simulink model "DockingApproachExample_Ext"  (Simulink 8.7)
settings: Solver=FixedStepDiscrete  StartTime=0.0  StopTime=300  RelTol=1e-3
libraries: simulink x2
settings Model: Creator=mwwhalen  LastModifiedBy=hamza
settings DataIOCC: ExternalInput=[t,u]  SaveFormat=Dataset  SignalLoggingSaveFormat=ModelDataLogs
settings OptimizationCC: ExpressionDepthLimit=2147483647  InitFltsAndDblsToZero=on
settings DebuggingCC: SaveWithParameterizedLinksMsg=none  SignalResolutionControl=TryResolveAllWithWarning  SolverPrmCheckMsg=warning  MultiTaskDSMMsg=warning  MultiTaskCondExecSysMsg=none  FcnCallInpInsideContextMsg=UseLocalSettings  StateNameClashWarn=warning
settings SFSimCC: SimParseCustomCode=off
settings RTWCC: PackageGeneratedCodeAndArtifacts=on  PackageName=DockingApproachExample_Ext_Code.zip  RTWCompilerOptimization=on
settings GRTTargetCC: TargetFcnLib=ansi_tfl_tmw.mat  CombineOutputUpdateFcns=off  GRTInterface=on

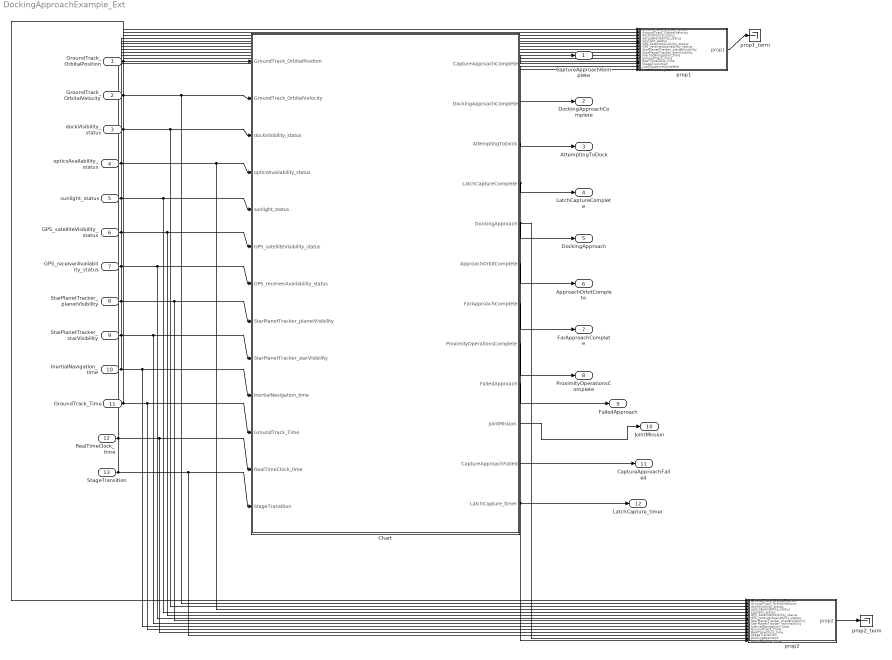
== system DockingApproachExample_Ext ==
  GroundTrack_OrbitalPosition : Inport
  GroundTrack_OrbitalVelocity : Inport  Port=2
  dockVisibility_status : Inport  Port=3
  opticsAvailability_status : Inport  Port=4
  sunlight_status : Inport  Port=5
  GPS_satelliteVisibility_status : Inport  Port=6
  GPS_receiverAvailability_status : Inport  Port=7
  StarPlanetTracker_planetVisibility : Inport  Port=8
  StarPlanetTracker_starVisibility : Inport  Port=9
  InertialNavigation_time : Inport  Port=10
  GroundTrack_Time : Inport  Port=11
  RealTimeClock_time : Inport  Port=12
  StageTransition : Inport  Port=13
  Chart : Stateflow chart  TreatAsAtomicUnit=on
  prop1 : Subsystem  TreatAsAtomicUnit=on  mask(Observer){AnnotationType=ensures, ObserverType=[]}
      mask prompts: AnnotationType "Type of annotation (pre/post...)"; ObserverType "Observer type"
      mask help:
      | Set an observer for the system.
      | The annotation type parameter sets the type of observer:
      | - requires : pre-condition
      | - ensures : post-condition
      | - assert : an assertion
      | - observer : the observer computes a special type of properties
      mask TypeOptions AnnotationType: ensures | requires | assert | observer
      mask Callback AnnotationType:
      | paramStr = get_param(gcb, 'MaskValues');
      | if strcmp(paramStr{1}(1),'o')
      | set_param(gcb,'MaskVisibilities',{'on';'on'});
      | paramStr{2} = 'ellipsoid';
      | set_param(gcb,'MaskValues',paramStr);
      | else
      | set_param(gcb,'MaskVisibilities',{'on';'off'});
      | end
      | clear paramStr;
      mask Callback ObserverType:
      | paramStr = get_param(gcb, 'MaskValues');
      | if strcmp(paramStr{1}(1),'o')
      | set_param(gcb,'MaskVisibilities',{'on';'on'});
      | paramStr{2} = 'ellipsoid';
      | set_param(gcb,'MaskValues',paramStr);
      | else
      | set_param(gcb,'MaskVisibilities',{'on';'off'});
      | end
      | clear paramStr;
      mask Display:
      | color('red')
      | text(0.5, 0.5, ['CoCoSpec: ''' get_param(gcb,'name') ''''], 'horizontalAlignment', 'center');
      | text(0.99, 0.03, '{\bf\fontsize{12}TO BE VERIFIED}', 'hor', 'right', 'ver', 'bottom', 'texmode', 'on');
  prop1_term : Terminator
  prop2 : Subsystem  TreatAsAtomicUnit=on  mask(Observer){AnnotationType=ensures, ObserverType=[]}
      mask prompts: AnnotationType "Type of annotation (pre/post...)"; ObserverType "Observer type"
      mask help:
      | Set an observer for the system.
      | The annotation type parameter sets the type of observer:
      | - requires : pre-condition
      | - ensures : post-condition
      | - assert : an assertion
      | - observer : the observer computes a special type of properties
      mask TypeOptions AnnotationType: ensures | requires | assert | observer
      mask Callback AnnotationType:
      | paramStr = get_param(gcb, 'MaskValues');
      | if strcmp(paramStr{1}(1),'o')
      | set_param(gcb,'MaskVisibilities',{'on';'on'});
      | paramStr{2} = 'ellipsoid';
      | set_param(gcb,'MaskValues',paramStr);
      | else
      | set_param(gcb,'MaskVisibilities',{'on';'off'});
      | end
      | clear paramStr;
      mask Callback ObserverType:
      | paramStr = get_param(gcb, 'MaskValues');
      | if strcmp(paramStr{1}(1),'o')
      | set_param(gcb,'MaskVisibilities',{'on';'on'});
      | paramStr{2} = 'ellipsoid';
      | set_param(gcb,'MaskValues',paramStr);
      | else
      | set_param(gcb,'MaskVisibilities',{'on';'off'});
      | end
      | clear paramStr;
      mask Display:
      | color('red')
      | text(0.5, 0.5, ['CoCoSpec: ''' get_param(gcb,'name') ''''], 'horizontalAlignment', 'center');
      | text(0.99, 0.03, '{\bf\fontsize{12}TO BE VERIFIED}', 'hor', 'right', 'ver', 'bottom', 'texmode', 'on');
  prop2_term : Terminator
  CaptureApproachComplete : Outport
  DockingApproachComplete : Outport  Port=2
  AttemptingToDock : Outport  Port=3
  LatchCaptureComplete : Outport  Port=4
  DockingApproach : Outport  Port=5
  ApproachOrbitComplete : Outport  Port=6
  FarApproachComplete : Outport  Port=7
  ProximityOperationsComplete : Outport  Port=8
  FailedApproach : Outport  Port=9
  JointMission : Outport  Port=10
  CaptureApproachFailed : Outport  Port=11
  LatchCapture_timer : Outport  Port=12
  wires:
  GroundTrack_OrbitalVelocity/1 -> Chart/2(GroundTrack_OrbitalVelocity), prop2/2(GroundTrack_OrbitalVelocity), prop1/2(GroundTrack_OrbitalVelocity)
  dockVisibility_status/1 -> Chart/3(dockVisibility_status), prop2/3(dockVisibility_status), prop1/3(dockVisibility_status)
  opticsAvailability_status/1 -> Chart/4(opticsAvailability_status), prop2/4(opticsAvailability_status), prop1/4(opticsAvailability_status)
  sunlight_status/1 -> Chart/5(sunlight_status), prop2/5(sunlight_status), prop1/5(sunlight_status)
  GPS_satelliteVisibility_status/1 -> Chart/6(GPS_satelliteVisibility_status), prop2/6(GPS_satelliteVisibility_status), prop1/6(GPS_satelliteVisibility_status)
  StarPlanetTracker_planetVisibility/1 -> Chart/8(StarPlanetTracker_planetVisibility), prop2/8(StarPlanetTracker_planetVisibility), prop1/8(StarPlanetTracker_planetVisibility)
  StarPlanetTracker_starVisibility/1 -> Chart/9(StarPlanetTracker_starVisibility), prop2/9(StarPlanetTracker_starVisibility), prop1/9(StarPlanetTracker_starVisibility)
  InertialNavigation_time/1 -> Chart/10(InertialNavigation_time), prop2/10(InertialNavigation_time), prop1/10(InertialNavigation_time)
  GroundTrack_Time/1 -> Chart/11(GroundTrack_Time), prop2/11(GroundTrack_Time), prop1/11(GroundTrack_Time)
  RealTimeClock_time/1 -> Chart/12(RealTimeClock_time), prop2/12(RealTimeClock_time), prop1/12(RealTimeClock_time)
  GroundTrack_OrbitalPosition/1 -> Chart/1(GroundTrack_OrbitalPosition), prop1/1(GroundTrack_OrbitalPosition), prop2/1(GroundTrack_OrbitalPosition)
  StageTransition/1 -> Chart/13(StageTransition), prop2/13(StageTransition), prop1/13(StageTransition)
  GPS_receiverAvailability_status/1 -> Chart/7(GPS_receiverAvailability_status), prop2/7(GPS_receiverAvailability_status), prop1/7(GPS_receiverAvailability_status)
  Chart/2(DockingApproachComplete) -> DockingApproachComplete/1
  Chart/1(CaptureApproachComplete) -> CaptureApproachComplete/1
  Chart/3(AttemptingToDock) -> AttemptingToDock/1
  Chart/4(LatchCaptureComplete) -> LatchCaptureComplete/1, prop1/14(LatchCaptureComplete)
  Chart/5(DockingApproach) -> DockingApproach/1, prop2/14(DockingApproach)
  Chart/6(ApproachOrbitComplete) -> ApproachOrbitComplete/1
  Chart/7(FarApproachComplete) -> FarApproachComplete/1
  Chart/8(ProximityOperationsComplete) -> ProximityOperationsComplete/1
  Chart/9(FailedApproach) -> FailedApproach/1
  Chart/10(JointMission) -> JointMission/1
  Chart/11(CaptureApproachFailed) -> CaptureApproachFailed/1
  Chart/12(LatchCapture_timer) -> LatchCapture_timer/1, prop1/15(LatchCapture_timer), prop2/15(LatchCapture_timer)
  prop1/1(prop1) -> prop1_term/1
  prop2/1(prop2) -> prop2_term/1

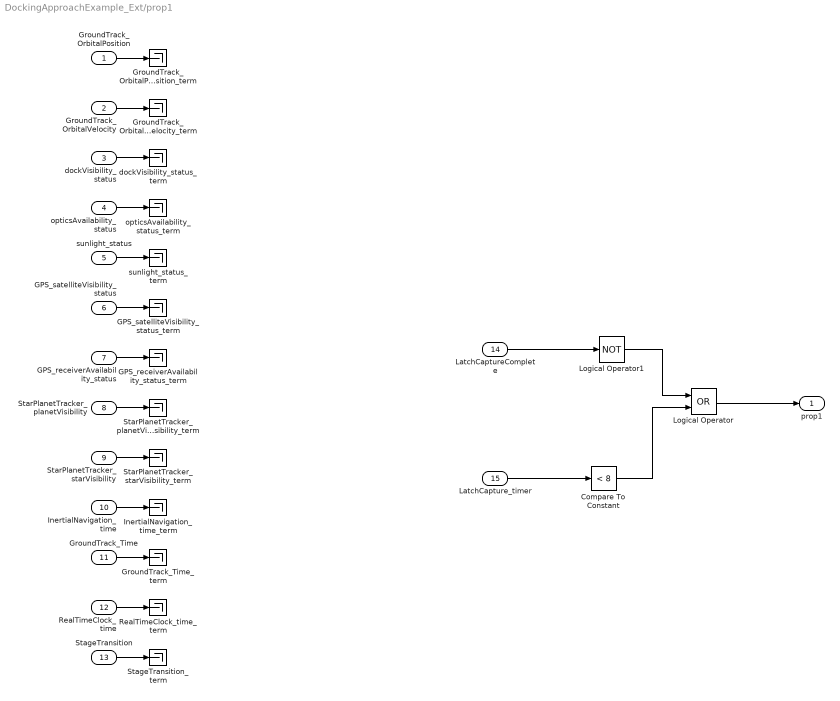
== system DockingApproachExample_Ext/prop1 ==
  GroundTrack_OrbitalPosition : Inport
  GroundTrack_OrbitalVelocity : Inport  Port=2
  dockVisibility_status : Inport  Port=3
  opticsAvailability_status : Inport  Port=4
  sunlight_status : Inport  Port=5
  GPS_satelliteVisibility_status : Inport  Port=6
  GPS_receiverAvailability_status : Inport  Port=7
  StarPlanetTracker_planetVisibility : Inport  Port=8
  StarPlanetTracker_starVisibility : Inport  Port=9
  InertialNavigation_time : Inport  Port=10
  GroundTrack_Time : Inport  Port=11
  RealTimeClock_time : Inport  Port=12
  StageTransition : Inport  Port=13
  LatchCaptureComplete : Inport  Port=14
  LatchCapture_timer : Inport  Port=15
  Compare To Constant : simulink/Logic and Bit Operations/Compare To Constant  relop=<  const=8  OutDataTypeStr=boolean
  GPS_receiverAvailability_status_term : Terminator
  GPS_satelliteVisibility_status_term : Terminator
  GroundTrack_OrbitalPosition_term : Terminator
  GroundTrack_OrbitalVelocity_term : Terminator
  GroundTrack_Time_term : Terminator
  InertialNavigation_time_term : Terminator
  Logical Operator : Logic  Operator=OR  AllPortsSameDT=off  OutDataTypeStr=boolean
  Logical Operator1 : Logic  Operator=NOT  AllPortsSameDT=off  OutDataTypeStr=boolean
  RealTimeClock_time_term : Terminator
  StageTransition_term : Terminator
  StarPlanetTracker_planetVisibility_term : Terminator
  StarPlanetTracker_starVisibility_term : Terminator
  dockVisibility_status_term : Terminator
  opticsAvailability_status_term : Terminator
  sunlight_status_term : Terminator
  prop1 : Outport
  wires:
  GroundTrack_OrbitalPosition/1 -> GroundTrack_OrbitalPosition_term/1
  GroundTrack_OrbitalVelocity/1 -> GroundTrack_OrbitalVelocity_term/1
  dockVisibility_status/1 -> dockVisibility_status_term/1
  opticsAvailability_status/1 -> opticsAvailability_status_term/1
  sunlight_status/1 -> sunlight_status_term/1
  GPS_satelliteVisibility_status/1 -> GPS_satelliteVisibility_status_term/1
  GPS_receiverAvailability_status/1 -> GPS_receiverAvailability_status_term/1
  StarPlanetTracker_planetVisibility/1 -> StarPlanetTracker_planetVisibility_term/1
  StarPlanetTracker_starVisibility/1 -> StarPlanetTracker_starVisibility_term/1
  InertialNavigation_time/1 -> InertialNavigation_time_term/1
  GroundTrack_Time/1 -> GroundTrack_Time_term/1
  RealTimeClock_time/1 -> RealTimeClock_time_term/1
  StageTransition/1 -> StageTransition_term/1
  LatchCaptureComplete/1 -> Logical Operator1/1
  LatchCapture_timer/1 -> Compare To Constant/1
  Logical Operator1/1 -> Logical Operator/1
  Compare To Constant/1 -> Logical Operator/2
  Logical Operator/1 -> prop1/1

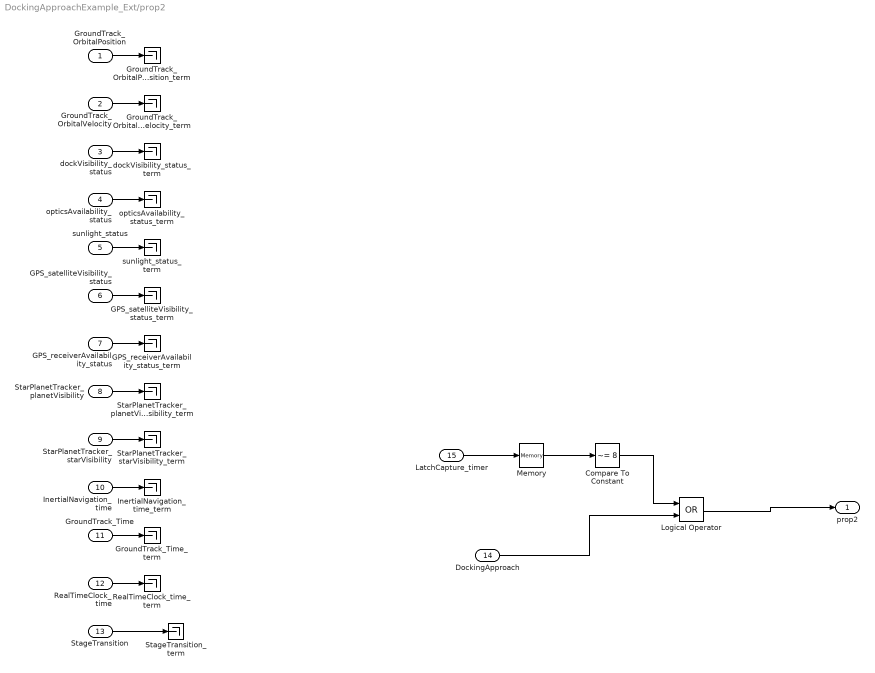
== system DockingApproachExample_Ext/prop2 ==
  GroundTrack_OrbitalPosition : Inport
  GroundTrack_OrbitalVelocity : Inport  Port=2
  dockVisibility_status : Inport  Port=3
  opticsAvailability_status : Inport  Port=4
  sunlight_status : Inport  Port=5
  GPS_satelliteVisibility_status : Inport  Port=6
  GPS_receiverAvailability_status : Inport  Port=7
  StarPlanetTracker_planetVisibility : Inport  Port=8
  StarPlanetTracker_starVisibility : Inport  Port=9
  InertialNavigation_time : Inport  Port=10
  GroundTrack_Time : Inport  Port=11
  RealTimeClock_time : Inport  Port=12
  StageTransition : Inport  Port=13
  DockingApproach : Inport  Port=14
  LatchCapture_timer : Inport  Port=15
  Compare To Constant : simulink/Logic and Bit Operations/Compare To Constant  relop=~=  const=8  OutDataTypeStr=boolean
  GPS_receiverAvailability_status_term : Terminator
  GPS_satelliteVisibility_status_term : Terminator
  GroundTrack_OrbitalPosition_term : Terminator
  GroundTrack_OrbitalVelocity_term : Terminator
  GroundTrack_Time_term : Terminator
  InertialNavigation_time_term : Terminator
  Logical Operator : Logic  Operator=OR  AllPortsSameDT=off  OutDataTypeStr=boolean
  Memory : Memory
  RealTimeClock_time_term : Terminator
  StageTransition_term : Terminator
  StarPlanetTracker_planetVisibility_term : Terminator
  StarPlanetTracker_starVisibility_term : Terminator
  dockVisibility_status_term : Terminator
  opticsAvailability_status_term : Terminator
  sunlight_status_term : Terminator
  prop2 : Outport
  wires:
  GroundTrack_OrbitalPosition/1 -> GroundTrack_OrbitalPosition_term/1
  GroundTrack_OrbitalVelocity/1 -> GroundTrack_OrbitalVelocity_term/1
  dockVisibility_status/1 -> dockVisibility_status_term/1
  opticsAvailability_status/1 -> opticsAvailability_status_term/1
  sunlight_status/1 -> sunlight_status_term/1
  GPS_satelliteVisibility_status/1 -> GPS_satelliteVisibility_status_term/1
  GPS_receiverAvailability_status/1 -> GPS_receiverAvailability_status_term/1
  StarPlanetTracker_planetVisibility/1 -> StarPlanetTracker_planetVisibility_term/1
  StarPlanetTracker_starVisibility/1 -> StarPlanetTracker_starVisibility_term/1
  InertialNavigation_time/1 -> InertialNavigation_time_term/1
  GroundTrack_Time/1 -> GroundTrack_Time_term/1
  RealTimeClock_time/1 -> RealTimeClock_time_term/1
  StageTransition/1 -> StageTransition_term/1
  DockingApproach/1 -> Logical Operator/2
  LatchCapture_timer/1 -> Memory/1
  Memory/1 -> Compare To Constant/1
  Compare To Constant/1 -> Logical Operator/1
  Logical Operator/1 -> prop2/1

== stateflow chart Chart ==
  settings: updateMethod=DISCRETE  sampleTime=1
  state fuel [parallel]
    settings: executionOrder=3
  state thrust [parallel]
    settings: executionOrder=2
    state y = compute(missionstate) [function]
      (default) -> (junction 74) : {}
    state y = command [function]
      (default) -> (junction 77) : {}
  state MissionPhaseStates [parallel]
    settings: executionOrder=1
    state FarApproach
    state JointStabilize
    state Start /
    state CollisionAvoidanceManuever/
      exit:
      ApproachOrbitComplete=0;
      ProximityOperationsComplete=0;
      FarApproachComplete=0;
      CaptureApproachComplete= 0;
    state FailedApproach /
      entry: FailedApproach=1;
    state ApproachOrbit
    state Disengage
    state ProximityOperations
    state JointMission /
      entry: JointMission=1;
    state DockingApproach/
      entry:
      DockingApproach = 1;
      DockingApproachComplete= 0;
      exit:
      DockingApproach = 0;
      state DockingApproach / [parallel]
        during :DockingApproach_timer = min(DockingApproach_timer+1,DockingApproach_timer_upper_limit/*9*/);
        settings: executionOrder=1
        note: This condition is our approximation
            | of missionState [GOOD]
        note: This condition is our approximation
            | of missionState [POOR]
        state StartApproach/
          entry : DockingApproach_timer = 0;
        state CheckTargetRelativeState
          /* missionState.compute (...) */
        state ReadyToDock/
          exit:
          DockingApproachComplete= 1;
        state ComputeThrust
        state DockingApproachFailed
        StartApproach -> CheckTargetRelativeState [order 1] : [dockingSensor_RelativePosition != NONE && ...
            | dockingSensor_RelativeVelocity != NONE && ...
            |  dockingSensor_RelativeAttitude != NONE &&...
            |  (DockingApproach_timer < DockingApproach_timer_upper_limit/*9*/)]
        (default) -> StartApproach
        StartApproach -> DockingApproachFailed [order 2] : [(DockingApproach_timer == DockingApproach_timer_upper_limit/*9*/)]
        CheckTargetRelativeState -> DockingApproachFailed [order 5] : [dockingSensor_targetState != GOOD]
        CheckTargetRelativeState -> DockingApproachFailed [order 4] : [dockingSensor_RelativePosition == NONE || ...
            | dockingSensor_RelativeVelocity == NONE || ...
            | dockingSensor_RelativeAttitude == NONE]
        CheckTargetRelativeState -> ReadyToDock [order 1] : [ dockingSensor_RelativePosition == GOOD &&...
            |   dockingSensor_RelativeVelocity == GOOD &...
            |   dockingSensor_RelativeAttitude == GOOD &&...
            |   dockingSensor_targetState == GOOD
            | /* MissionState_status == GOOD */ ]
        CheckTargetRelativeState -> DockingApproachFailed [order 3] : [(DockingApproach_timer == DockingApproach_timer_upper_limit/*9*/)]
        ComputeThrust -> CheckTargetRelativeState [order 1] : [thrust_status == EXIST && ...
            | fuel_status == GOOD]
        CheckTargetRelativeState -> ComputeThrust [order 2] : [ dockingSensor_RelativePosition == POOR &&...
            |   dockingSensor_RelativeVelocity == POOR &&...
            |   dockingSensor_RelativeAttitude == POOR &&...
            |   dockingSensor_targetState == POOR
            | /* MissionState_status == POOR */]
        ComputeThrust -> DockingApproachFailed [order 2] : [!(thrust_status == EXIST && ...
            |  fuel_status == GOOD)||...
            | DockingApproach_timer == DockingApproach_timer_upper_limit]
      state dockingSensor / [parallel]
        during:dockingSensor_timer = min(dockingSensor_timer + 1,dockingSensor_timer_upper_limit/*6*/);
        settings: executionOrder=2
        state Good /
          entry : dockingSensor_RelativePosition = GOOD;
          dockingSensor_RelativeVelocity = GOOD;
          dockingSensor_RelativeAttitude = GOOD;
          dockingSensor_targetState = GOOD;
          exit :  dockingSensor_timer = 0;
        state Poor /
          entry :dockingSensor_RelativePosition = POOR;
          dockingSensor_RelativeVelocity = POOR;
          dockingSensor_RelativeAttitude = POOR;
          dockingSensor_targetState = POOR;
        state Acquiring /
          entry : dockingSensor_RelativePosition = NONE;
          dockingSensor_RelativeVelocity = NONE;
          dockingSensor_RelativeAttitude = NONE;
          dockingSensor_targetState = NONE;
          exit :  dockingSensor_timer = 0;
        (default) -> MissionPhaseStates.DockingApproach.dockingSensor.Acquiring 
        Poor  -> MissionPhaseStates.DockingApproach.dockingSensor.Acquiring  [order 1] : [(dockingSensor_timer == dockingSensor_timer_upper_limit/*6*/) && ...
            | (dockVisibility_status == NONE || ...
            | opticsAvailability_status != AVAILABLE)]
        MissionPhaseStates.DockingApproach.dockingSensor.Acquiring  -> Poor  [order 1] : [dockVisibility_status != NONE && ...
            | opticsAvailability_status == AVAILABLE]
        MissionPhaseStates.DockingApproach.dockingSensor.Acquiring  -> MissionPhaseStates.DockingApproach.dockingSensor.Acquiring  [order 2] : [dockVisibility_status == NONE || ...
            | opticsAvailability_status != AVAILABLE]
        Poor  -> Poor  [order 3] : [(dockingSensor_timer < dockingSensor_timer_upper_limit/*6*/) &&...
            | (dockVisibility_status == NONE || ...
            | opticsAvailability_status != AVAILABLE)||...
            | (opticsAvailability_status == AVAILABLE &&...
            | (dockVisibility_status == POOR || ...
            | sunlight_status == BRIGHT))]
        Good  -> Poor  [order 1] : [(dockVisibility_status != GOOD && ...
            | opticsAvailability_status != AVAILABLE) || ...
            | sunlight_status == BRIGHT]
        Poor  -> Good  [order 2] : [(dockingSensor_timer < dockingSensor_timer_upper_limit) /* or ==6? */&&...
            | dockVisibility_status == GOOD && ...
            | opticsAvailability_status == AVAILABLE && ...
            | sunlight_status != BRIGHT]
        Good  -> Good  [order 2] : [dockVisibility_status == GOOD && ...
            | opticsAvailability_status == AVAILABLE && ...
            | sunlight_status != BRIGHT]
    state CaptureApproach /
      state CaptureApproach/ [parallel]
        during:CaptureApproach_timer = min(CaptureApproach_timer+1,CaptureApproach_timer_upper_limit)
        settings: executionOrder=1
        state StartApproach /
          entry :  CaptureApproach_timer = 0;
          CaptureApproachFailed = 0;
        state CheckOrbitalState
        state ComputeThrust /
          entry : /*thrust.compute(...
          CaptureMissionState)*/
        state OrientedForDockingApproach/
          exit:
          CaptureApproachComplete= 1;
        state CaptureApproachFailed /
          entry: CaptureApproachFailed = 1;
        (default) -> StartApproach 
        StartApproach  -> CheckOrbitalState [order 1] : [ OrbitalState_Position != NONE &&...
            |   OrbitalState_Velocity != NONE &&...
            |   OrbitalState_Attitude != NONE && ...
            |   OrbitalState_Time != NONE &&...
            |  (CaptureApproach_timer < CaptureApproach_timer_upper_limit)]
        StartApproach  -> CaptureApproachFailed  [order 2] : [CaptureApproach_timer ==...
            | CaptureApproach_timer_upper_limit]
        CheckOrbitalState -> OrientedForDockingApproach [order 1] : [OrbitalState_Position == GOOD...
            |  &&...
            |  OrbitalState_Velocity == GOOD...
            |  &&...
            |  OrbitalState_Attitude != NONE...
            |   &&...
            |  OrbitalState_Time == GOOD]
        ComputeThrust  -> CheckOrbitalState [order 1] : [thrust_status == EXIST &&...
            |  fuel_status == GOOD]
        CheckOrbitalState -> ComputeThrust  [order 2] : [OrbitalState_Position == POOR...
            |  &&...
            |  OrbitalState_Velocity == POOR...
            |  &&...
            |  OrbitalState_Attitude == NONE...
            |   &&...
            |  OrbitalState_Time == POOR]
        CheckOrbitalState -> CaptureApproachFailed  [order 3] : [(OrbitalState_Position == NONE ||...
            | OrbitalState_Velocity == NONE || ...
            | OrbitalState_Attitude == NONE ||...
            |  OrbitalState_Time == NONE) ||...
            |  (CaptureApproach_timer == ...
            | CaptureApproach_timer_upper_limit)]
        ComputeThrust  -> CaptureApproachFailed  [order 2] : [!(thrust_status == EXIST &&...
            | fuel_status == GOOD) || (CaptureApproach_timer == CaptureApproach_timer_upper_limit)]
      state OrbitalState_Active/ [parallel]
        settings: executionOrder=2
        state OrbitalState_Complex / [parallel]
          settings: executionOrder=1
          state OrbitalState/ [parallel]
            settings: executionOrder=1
            state Acquiring /
              entry : OrbitalState_Position = NONE;
              OrbitalState_Velocity = NONE;
              OrbitalState_Attitude = NONE;
            state POOR /
              entry : OrbitalState_Position = POOR;
              OrbitalState_Velocity = POOR;
              OrbitalState_Attitude = NONE;
            state pvGOOD /
              entry : OrbitalState_Position = GOOD;
              OrbitalState_Velocity = GOOD;
              OrbitalState_Attitude = POOR;
            state GOOD /
              entry : OrbitalState_Position = GOOD;
              OrbitalState_Velocity = GOOD;
              OrbitalState_Attitude = GOOD;
            MissionPhaseStates.CaptureApproach.OrbitalState_Active.OrbitalState_Complex.OrbitalState.Acquiring  -> MissionPhaseStates.CaptureApproach.OrbitalState_Active.OrbitalState_Complex.OrbitalState.Acquiring  [order 2] : [GPS_AbsolutePosition == NONE && GPS_AbsoluteVelocity == NONE && ...
                | StarPlanetTracker_AbsolutePosition == NONE && ...
                | StarPlanetTracker_AbsoluteVelocity == NONE &&...
                | GroundTrack_OrbitalPosition == NONE&&...
                | GroundTrack_OrbitalVelocity == NONE]
            (default) -> MissionPhaseStates.CaptureApproach.OrbitalState_Active.OrbitalState_Complex.OrbitalState.Acquiring 
            MissionPhaseStates.CaptureApproach.OrbitalState_Active.OrbitalState_Complex.OrbitalState.POOR  -> MissionPhaseStates.CaptureApproach.OrbitalState_Active.OrbitalState_Complex.OrbitalState.Acquiring  [order 1] : [(GroundTrack_OrbitalPosition == NONE &&...
                | GPS_AbsolutePosition == NONE &&...
                | StarPlanetTracker_AbsolutePosition == NONE) &&...
                | (GroundTrack_OrbitalVelocity == NONE &&...
                | GPS_AbsoluteVelocity == NONE &&...
                | StarPlanetTracker_AbsoluteVelocity == NONE)]
            MissionPhaseStates.CaptureApproach.OrbitalState_Active.OrbitalState_Complex.OrbitalState.Acquiring  -> MissionPhaseStates.CaptureApproach.OrbitalState_Active.OrbitalState_Complex.OrbitalState.POOR  [order 1] : [!(GPS_AbsolutePosition == NONE &&...
                |  StarPlanetTracker_AbsolutePosition == NONE&&...
                | GroundTrack_OrbitalPosition == NONE)&&...
                | !(GPS_AbsoluteVelocity == NONE &&...
                |  StarPlanetTracker_AbsoluteVelocity == NONE&&...
                | GroundTrack_OrbitalVelocity == NONE)]
            MissionPhaseStates.CaptureApproach.OrbitalState_Active.OrbitalState_Complex.OrbitalState.POOR  -> (junction 140) [order 2] : [((GroundTrack_OrbitalPosition == GOOD && ...
                |   GPS_AbsolutePosition == GOOD)|| ...
                |   (GroundTrack_OrbitalPosition == GOOD &&...
                | StarPlanetTracker_AbsolutePosition == GOOD)||...
                | (StarPlanetTracker_AbsolutePosition == GOOD &&...
                |  GPS_AbsolutePosition == GOOD)||...
                |  (InertialNavigation_AbsolutePosition == GOOD&&...
                |  GroundTrack_OrbitalPosition == GOOD)||...
                | (InertialNavigation_AbsolutePosition == GOOD&&...
                | GPS_AbsolutePosition == GOOD)|| ...
                | (InertialNavigation_AbsolutePosition == GOOD&&...
                |  StarPlanetTracker_AbsolutePosition == GOOD))]
            (junction 141) -> MissionPhaseStates.CaptureApproach.OrbitalState_Active.OrbitalState_Complex.OrbitalState.POOR  : [!((GroundTrack_OrbitalVelocity == GOOD && ...
                |   GPS_AbsoluteVelocity == GOOD)|| ...
                |   (GroundTrack_OrbitalVelocity == GOOD &&...
                | StarPlanetTracker_AbsoluteVelocity == GOOD)||...
                | (StarPlanetTracker_AbsoluteVelocity == GOOD &&...
                |  GPS_AbsoluteVelocity == GOOD)||...
                | (InertialNavigation_AbsoluteVelocity == GOOD&&...
                |  GroundTrack_OrbitalVelocity == GOOD)||...
                | (InertialNavigation_AbsoluteVelocity == GOOD&&...
                | GPS_AbsoluteVelocity == GOOD)|| ...
                | (InertialNavigation_AbsoluteVelocity == GOOD&&...
                |  StarPlanetTracker_AbsoluteVelocity == GOOD))]
            (junction 140) -> (junction 142) : [((GroundTrack_OrbitalVelocity == GOOD && ...
                |   GPS_AbsoluteVelocity == GOOD)|| ...
                |   (GroundTrack_OrbitalVelocity == GOOD &&...
                | StarPlanetTracker_AbsoluteVelocity == GOOD)||...
                | (StarPlanetTracker_AbsoluteVelocity == GOOD &&...
                |  GPS_AbsoluteVelocity == GOOD)||...
                | (InertialNavigation_AbsoluteVelocity == GOOD&&...
                |  GroundTrack_OrbitalVelocity == GOOD)||...
                | (InertialNavigation_AbsoluteVelocity == GOOD&&...
                | GPS_AbsoluteVelocity == GOOD)|| ...
                | (InertialNavigation_AbsoluteVelocity == GOOD&&...
                |  StarPlanetTracker_AbsoluteVelocity == GOOD))]
            (junction 143) -> (junction 141) : [!(InertialNavigation_AbsoluteAttitude == GOOD||...
                | StarPlanetTracker_AbsoluteAttitude == GOOD)]
            (junction 142) -> pvGOOD  : [InertialNavigation_AbsoluteAttitude == GOOD||...
                | StarPlanetTracker_AbsoluteAttitude == GOOD]
            MissionPhaseStates.CaptureApproach.OrbitalState_Active.OrbitalState_Complex.OrbitalState.GOOD  -> (junction 143) [order 1] : [!((GroundTrack_OrbitalPosition == GOOD && ...
                |   GPS_AbsolutePosition == GOOD)|| ...
                |   (GroundTrack_OrbitalPosition == GOOD &&...
                | StarPlanetTracker_AbsolutePosition == GOOD)||...
                | (StarPlanetTracker_AbsolutePosition == GOOD &&...
                |  GPS_AbsolutePosition == GOOD)||...
                |  (InertialNavigation_AbsolutePosition == GOOD&&...
                |  GroundTrack_OrbitalPosition == GOOD)||...
                | (InertialNavigation_AbsolutePosition == GOOD&&...
                | GPS_AbsolutePosition == GOOD)|| ...
                | (InertialNavigation_AbsolutePosition == GOOD&&...
                |  StarPlanetTracker_AbsolutePosition == GOOD))]
            pvGOOD  -> MissionPhaseStates.CaptureApproach.OrbitalState_Active.OrbitalState_Complex.OrbitalState.GOOD  : [(GroundTrack_OrbitalPosition == GOOD || ...
                | GPS_AbsolutePosition == GOOD || ...
                | StarPlanetTracker_AbsolutePosition == GOOD)...
                |  && (GroundTrack_OrbitalVelocity == GOOD || ...
                | GPS_AbsoluteVelocity == GOOD || ...
                | StarPlanetTracker_AbsoluteVelocity == GOOD)...
                | && StarPlanetTracker_AbsoluteAttitude == GOOD]/
                | /*send(callibrate,InertialNavigation)*/
            MissionPhaseStates.CaptureApproach.OrbitalState_Active.OrbitalState_Complex.OrbitalState.GOOD  -> MissionPhaseStates.CaptureApproach.OrbitalState_Active.OrbitalState_Complex.OrbitalState.GOOD  [order 2] : [(GroundTrack_OrbitalPosition == GOOD || ...
                | GPS_AbsolutePosition == GOOD || ...
                | StarPlanetTracker_AbsolutePosition == GOOD)...
                |  && (GroundTrack_OrbitalVelocity == GOOD || ...
                | GPS_AbsoluteVelocity == GOOD || ...
                | StarPlanetTracker_AbsoluteVelocity == GOOD)...
                | && StarPlanetTracker_AbsoluteAttitude == GOOD]/
                | /*send(callibrate,InertialNavigation)*/
          state y = RealTimeClock_callibrate [function]
            (default) -> (junction 157) : {}
          state OrbitalState2 / [parallel]
            settings: executionOrder=2
            state POOR/
              entry : OrbitalState_Time = POOR
            state GOOD /
              entry : OrbitalState_Time = GOOD
            (default) -> MissionPhaseStates.CaptureApproach.OrbitalState_Active.OrbitalState_Complex.OrbitalState2.POOR
            MissionPhaseStates.CaptureApproach.OrbitalState_Active.OrbitalState_Complex.OrbitalState2.GOOD  -> MissionPhaseStates.CaptureApproach.OrbitalState_Active.OrbitalState_Complex.OrbitalState2.POOR [order 1] : [RealTimeClock_time != GOOD]
            MissionPhaseStates.CaptureApproach.OrbitalState_Active.OrbitalState_Complex.OrbitalState2.POOR -> MissionPhaseStates.CaptureApproach.OrbitalState_Active.OrbitalState_Complex.OrbitalState2.GOOD  : [GroundTrack_Time== GOOD...
                | || GPS_AbsoluteTime == GOOD || ...
                | StarPlanetTracker_AbsoluteTime == GOOD]
            MissionPhaseStates.CaptureApproach.OrbitalState_Active.OrbitalState_Complex.OrbitalState2.GOOD  -> MissionPhaseStates.CaptureApproach.OrbitalState_Active.OrbitalState_Complex.OrbitalState2.GOOD  [order 2] : [GroundTrack_Time == GOOD...
                | || GPS_AbsoluteTime == GOOD || ...
                | StarPlanetTracker_AbsoluteTime == GOOD]...
                | /*/RealTimeClock_callibrate()*/
        state GPS / [parallel]
          during:GPS_timer = min(GPS_timer + 1,GPS_timer_upper_limit/*6*/);
          settings: executionOrder=2
          state ACQUIRING /
            entry : GPS_AbsolutePosition = NONE;
            GPS_AbsoluteVelocity = NONE;
            GPS_AbsoluteTime = NONE;
          state POOR /
            entry : GPS_timer = 0;
            GPS_AbsolutePosition = POOR;
            GPS_AbsoluteVelocity = POOR;
            GPS_AbsoluteTime = POOR;
          state GOOD /
            entry : GPS_AbsolutePosition = GOOD;
            GPS_AbsoluteVelocity = GOOD;
            GPS_AbsoluteTime = GOOD;
          MissionPhaseStates.CaptureApproach.OrbitalState_Active.GPS.POOR  -> MissionPhaseStates.CaptureApproach.OrbitalState_Active.GPS.ACQUIRING  [order 1] : [(GPS_timer == GPS_timer_upper_limit /*5*/) && (GPS_satelliteVisibility_status == NONE || ...
              | GPS_receiverAvailability_status != AVAILABLE)]
          (default) -> MissionPhaseStates.CaptureApproach.OrbitalState_Active.GPS.ACQUIRING 
          MissionPhaseStates.CaptureApproach.OrbitalState_Active.GPS.ACQUIRING  -> MissionPhaseStates.CaptureApproach.OrbitalState_Active.GPS.ACQUIRING  [order 2] : [GPS_satelliteVisibility_status == NONE || GPS_receiverAvailability_status != AVAILABLE]
          MissionPhaseStates.CaptureApproach.OrbitalState_Active.GPS.ACQUIRING  -> MissionPhaseStates.CaptureApproach.OrbitalState_Active.GPS.POOR  [order 1] : [GPS_satelliteVisibility_status != NONE && GPS_receiverAvailability_status == AVAILABLE]
          MissionPhaseStates.CaptureApproach.OrbitalState_Active.GPS.POOR  -> MissionPhaseStates.CaptureApproach.OrbitalState_Active.GPS.POOR  [order 3] : [(GPS_timer < GPS_timer_upper_limit /*6*/) && (GPS_satelliteVisibility_status == NONE || ...
              | GPS_receiverAvailability_status != AVAILABLE) || (GPS_receiverAvailability_status == AVAILABLE && ...
              | (GPS_satelliteVisibility_status == POOR || sunlight_status == BRIGHT))]
          MissionPhaseStates.CaptureApproach.OrbitalState_Active.GPS.POOR  -> MissionPhaseStates.CaptureApproach.OrbitalState_Active.GPS.GOOD  [order 2] : [(GPS_timer == GPS_timer_upper_limit /*5*/) && GPS_satelliteVisibility_status == GOOD && ...
              | GPS_receiverAvailability_status == AVAILABLE && sunlight_status != BRIGHT]
          MissionPhaseStates.CaptureApproach.OrbitalState_Active.GPS.GOOD  -> MissionPhaseStates.CaptureApproach.OrbitalState_Active.GPS.POOR  [order 1] : [!(GPS_satelliteVisibility_status == GOOD &&...
              | GPS_receiverAvailability_status == AVAILABLE) || ...
              | sunlight_status == BRIGHT]
          MissionPhaseStates.CaptureApproach.OrbitalState_Active.GPS.GOOD  -> MissionPhaseStates.CaptureApproach.OrbitalState_Active.GPS.GOOD  [order 2] : [GPS_satelliteVisibility_status == GOOD && GPS_receiverAvailability_status == AVAILABLE && ...
              | sunlight_status != BRIGHT]
        state StarPlanetTracker / [parallel]
          during:StarPlanetTracker_timer = min(StarPlanetTracker_timer + 1,StarPlanetTracker_timer_upper_limit/*6*/);
          settings: executionOrder=3
          state ACQUIRING /
            entry : StarPlanetTracker_AbsolutePosition = NONE;
            StarPlanetTracker_AbsoluteVelocity = NONE;
            StarPlanetTracker_AbsoluteAttitude = NONE;
            StarPlanetTracker_AbsoluteTime = NONE;
          state POOR /
            entry : StarPlanetTracker_timer = 0;
            StarPlanetTracker_AbsolutePosition = POOR;
            StarPlanetTracker_AbsoluteVelocity = POOR;
            StarPlanetTracker_AbsoluteAttitude  = POOR;
            StarPlanetTracker_AbsoluteTime = POOR;
          state GOOD /
            entry: StarPlanetTracker_AbsolutePosition = GOOD;
            StarPlanetTracker_AbsoluteVelocity = GOOD;
            StarPlanetTracker_AbsoluteAttitude = GOOD;
            StarPlanetTracker_AbsoluteTime = GOOD;
          (default) -> MissionPhaseStates.CaptureApproach.OrbitalState_Active.StarPlanetTracker.ACQUIRING 
          MissionPhaseStates.CaptureApproach.OrbitalState_Active.StarPlanetTracker.ACQUIRING  -> MissionPhaseStates.CaptureApproach.OrbitalState_Active.StarPlanetTracker.ACQUIRING  [order 2] : [StarPlanetTracker_planetVisibility == NONE ||...
              |  StarPlanetTracker_starVisibility == NONE || ...
              |  opticsAvailability_status != AVAILABLE]
          MissionPhaseStates.CaptureApproach.OrbitalState_Active.StarPlanetTracker.ACQUIRING  -> MissionPhaseStates.CaptureApproach.OrbitalState_Active.StarPlanetTracker.POOR  [order 1] : [!(StarPlanetTracker_planetVisibility == NONE ||...
              |  StarPlanetTracker_starVisibility == NONE) && ...
              |  opticsAvailability_status == AVAILABLE]
          MissionPhaseStates.CaptureApproach.OrbitalState_Active.StarPlanetTracker.POOR  -> MissionPhaseStates.CaptureApproach.OrbitalState_Active.StarPlanetTracker.ACQUIRING  [order 1] : [(StarPlanetTracker_timer ==...
              |  StarPlanetTracker_timer_upper_limit /*6*/) && ...
              |   (StarPlanetTracker_planetVisibility == NONE || ...
              |    StarPlanetTracker_starVisibility == NONE || ...
              |    opticsAvailability_status != AVAILABLE)]
          MissionPhaseStates.CaptureApproach.OrbitalState_Active.StarPlanetTracker.POOR  -> MissionPhaseStates.CaptureApproach.OrbitalState_Active.StarPlanetTracker.POOR  [order 3] : [ StarPlanetTracker_timer < StarPlanetTracker_timer_upper_limit  /*6 */&& ...
              |     (StarPlanetTracker_planetVisibility == NONE || ...
              |      StarPlanetTracker_starVisibility == NONE ||...
              |      opticsAvailability_status != AVAILABLE)  || ...
              |    (opticsAvailability_status == AVAILABLE &&...
              |      (sunlight_status == BRIGHT||...
              |       StarPlanetTracker_planetVisibility == POOR || ...
              |       StarPlanetTracker_starVisibility == POOR))]
          MissionPhaseStates.CaptureApproach.OrbitalState_Active.StarPlanetTracker.POOR  -> MissionPhaseStates.CaptureApproach.OrbitalState_Active.StarPlanetTracker.GOOD  [order 2] : [(StarPlanetTracker_timer == StarPlanetTracker_timer_upper_limit /* 6*/) &&...
              |  StarPlanetTracker_planetVisibility == GOOD && ...
              | StarPlanetTracker_starVisibility == GOOD &&...
              |  opticsAvailability_status == AVAILABLE && ...
              | sunlight_status != BRIGHT]
          MissionPhaseStates.CaptureApproach.OrbitalState_Active.StarPlanetTracker.GOOD  -> MissionPhaseStates.CaptureApproach.OrbitalState_Active.StarPlanetTracker.POOR  [order 1] : [(StarPlanetTracker_planetVisibility != GOOD &&...
              |  StarPlanetTracker_starVisibility != GOOD && ...
              | opticsAvailability_status != AVAILABLE ) ||...
              |  sunlight_status == BRIGHT]
          MissionPhaseStates.CaptureApproach.OrbitalState_Active.StarPlanetTracker.GOOD  -> MissionPhaseStates.CaptureApproach.OrbitalState_Active.StarPlanetTracker.GOOD  [order 2] : [StarPlanetTracker_planetVisibility == GOOD &&...
              |  StarPlanetTracker_starVisibility == GOOD && ...
              |  opticsAvailability_status == AVAILABLE && sunlight_status != BRIGHT]
        state InertialNavigation/ [parallel]
          during:InertialNavigation_timer = min(InertialNavigation_timer+1,InertialNavigation_timer_upper_limit/*6*/);
          settings: executionOrder=4
          state POOR/
            entry:InertialNavigation_AbsolutePosition = POOR;
            InertialNavigation_AbsoluteVelocity = POOR;
            InertialNavigation_AbsoluteAttitude = POOR;
          state ACQUIRING/
            entry:InertialNavigation_AbsolutePosition = NONE;
            InertialNavigation_AbsoluteVelocity = NONE;
            InertialNavigation_AbsoluteAttitude = NONE;
          state GOOD/
            entry:InertialNavigation_timer = 0;
            InertialNavigation_AbsolutePosition = GOOD;
            InertialNavigation_AbsoluteVelocity = GOOD;
            InertialNavigation_AbsoluteAttitude = GOOD;
          (default) -> ACQUIRING
          ACQUIRING -> GOOD : callibrate
          (junction 180) -> ACQUIRING : [InertialNavigation_time != VALID]
          MissionPhaseStates.CaptureApproach.OrbitalState_Active.InertialNavigation.POOR -> (junction 180) [order 2]
          GOOD -> (junction 180) [order 3]
          GOOD -> GOOD [order 2] : [InertialNavigation_timer < InertialNavigation_timer_upper_limit /*6*/]
          GOOD -> MissionPhaseStates.CaptureApproach.OrbitalState_Active.InertialNavigation.POOR [order 1] : [InertialNavigation_timer == InertialNavigation_timer_upper_limit /*6*/]
          MissionPhaseStates.CaptureApproach.OrbitalState_Active.InertialNavigation.POOR -> GOOD [order 1] : callibrate
    state LatchCapture
      state LatchCaptureCheck / [parallel]
        entry:AttemptingToDock = 1;
        during:LatchCapture_timer = min(LatchCapture_timer + 1,LatchCapture_timer_upper_limit+1/*9*/);
        exit : AttemptingToDock = 0;
        settings: executionOrder=1
        state CheckLatchOpen /
          entry : LatchCapture_timer = 0;
        state CheckLatchMated
        state LatchFailed
        state Docked
          entry:LatchCaptureComplete = 1;
        (default) -> CheckLatchOpen 
        CheckLatchOpen  -> CheckLatchMated [order 1] : [latch_status == OPEN]
        CheckLatchMated -> Docked [order 1] : [latch_status == MATED]
        CheckLatchMated -> (junction 191) [order 3] : [LatchCapture_timer == LatchCapture_timer_upper_limit/*9*/]
        CheckLatchMated -> (junction 191) [order 2] : [latch_status == CLOSEDBUTUNMATED]
        CheckLatchOpen  -> LatchFailed [order 2] : [LatchCapture_timer == LatchCapture_timer_upper_limit/*9*/]
        (junction 191) -> LatchFailed
      state latch [parallel]
        settings: executionOrder=2
        state Opening /
          entry : latch_status = INDETERMINATE
        state Open /
          entry : latch_status = OPEN
        state Closing /
          entry : latch_status = INDETERMINATE
        state Mated /
          entry : latch_status = MATED
        state ClosedButUnmated /
          entry : latch_status = CLOSEDBUTUNMATED
        (default) -> Opening 
        (junction 199) -> Opening 
        Opening  -> Closing  [order 2] : /*closeLatch*/
        Opening  -> Open  [order 1] : /*open*/
        Open  -> Closing  : /*closeLatch*/
        Closing  -> ClosedButUnmated  [order 3] : /*closedButUnmated*/
        Closing  -> Mated  [order 1] : /*mated*/
        Closing  -> (junction 199) [order 2] : /*openLatch*/
        Mated  -> (junction 199) : /*openLatch*/
        ClosedButUnmated  -> (junction 199)
    (default) -> Start 
    Start  -> ApproachOrbit : [StageTransition == 0
        | /*Approach*/]
    CollisionAvoidanceManuever -> ApproachOrbit [order 2] : [StageTransition == 6]
        | /*isSafeToApproach*/
    ProximityOperations -> ApproachOrbit [order 1] : [StageTransition == 1]
        | {ApproachOrbitComplete=0;}
        | /*FailedProximityApproach*/
    ApproachOrbit -> ProximityOperations : [StageTransition == 2]
        | {ApproachOrbitComplete=1}
        |  /*isInSameOrbit*/
    FarApproach -> CollisionAvoidanceManuever [order 1] : [StageTransition == 5]
        | /*FailedFarApproach*/
    Disengage -> CollisionAvoidanceManuever : [StageTransition == 7]
        | /*isDisengaged*/
    CollisionAvoidanceManuever -> FailedApproach  [order 1] : [StageTransition == 8]
        | /*FailedApproach*/
    ProximityOperations -> FarApproach [order 2] : [StageTransition == 3]
        | {ProximityOperationsComplete=1}
        | /*isInSight*/
    JointStabilize -> Disengage [order 1] : [ StageTransition == 9]
        | /*LatchLost*/
    FarApproach -> CaptureApproach  [order 2] : [StageTransition == 4]
        | {FarApproachComplete=1}
        | /*InProximity*/
    JointStabilize -> JointMission  [order 2] : [StageTransition == 10]
        | /*JointMission*/
    ReadyToDock -> LatchCapture : /*ReadyToDock*/
    DockingApproachFailed -> CheckOrbitalState : /*DockingApproachFailed*/
    CaptureApproachFailed  -> CollisionAvoidanceManuever : /*CaptureApproachFailed*/
    OrientedForDockingApproach -> DockingApproach : /*Oriented*/
    Docked -> JointStabilize : /*Docked*/
    LatchFailed -> CheckTargetRelativeState : /*LatchFailed*/
  data: missionstate function_input int8; y function_output int8; y function_output double; targetState local int8; y function_output uint32; VALID local boolean; INDETERMINATE constant int8; OPEN constant int8 =1; CLOSEDBUTUNMATED constant int8 =2; MATED constant int8 =3; EXIST constant int8 =1; AVAILABLE constant boolean =1; EXPIRED constant boolean =1; OrbitalState_Position local int8; OrbitalState_Velocity local int8; OrbitalState_Attitude local int8; OrbitalState_Time local int8; NONE constant int8; POOR constant int8 =1; GOOD constant int8 =2; InertialNavigation_AbsolutePosition local int8; InertialNavigation_AbsoluteAttitude local int8; InertialNavigation_AbsoluteVelocity local int8; GroundTrack_OrbitalPosition input int8; GPS_AbsoluteVelocity local int8; GPS_AbsoluteTime local int8; GroundTrack_OrbitalVelocity input int8; StarPlanetTracker_AbsoluteAttitude local int8; StarPlanetTracker_AbsolutePosition local int8; StarPlanetTracker_AbsoluteTime local int8; StarPlanetTracker_AbsoluteVelocity local int8; GPS_AbsolutePosition local int8; dockingSensor_RelativePosition local int8; dockingSensor_RelativeVelocity local int8; dockingSensor_RelativeAttitude local int8; dockingSensor_targetState local int8; thrust_status local int8; fuel_status local int8; DockingApproach_timer local int8; CaptureApproach_timer local int8; dockVisibility_status input int8; opticsAvailability_status input boolean; sunlight_status input boolean; GPS_satelliteVisibility_status input int8; GPS_receiverAvailability_status input boolean; StarPlanetTracker_planetVisibility input int8; StarPlanetTracker_starVisibility input int8; InertialNavigation_time input boolean; GroundTrack_Time input int8; latch_status local int8; dockingSensor_timer local int8; InertialNavigation_timer local int8; StarPlanetTracker_timer local int8; GPS_timer local int8; RealTimeClock_time input int8; BRIGHT constant boolean =1; StageTransition input int8; CaptureApproach_timer_upper_limit constant int8 =11; CaptureApproachComplete output boolean; DockingApproachComplete output boolean; AttemptingToDock output boolean; LatchCaptureComplete output boolean; DockingApproach output boolean; ApproachOrbitComplete output boolean; FarApproachComplete output boolean; ProximityOperationsComplete output boolean; FailedApproach output boolean; JointMission output boolean; StarPlanetTracker_timer_upper_limit constant int8 =6; InertialNavigation_timer_upper_limit constant int8 =6; DockingApproach_timer_upper_limit constant int8 =9; dockingSensor_timer_upper_limit constant int8 =6; CaptureApproachFailed output boolean; LatchCapture_timer output int8; GPS_timer_upper_limit constant int8 =6; LatchCapture_timer_upper_limit constant int8 =8
  events: callibrate local EITHER_EDGE_EVENT
